simulink model "MassSpringModel"  (R2015b)
settings: Solver=ode1  StartTime=0.0  StopTime=10.0  FixedStep=0.0001  RelTol=1e-3
model workspace (MAT data in the model file):
  ans = 35
  c = 1.7
  d = 1
  g = 9.81
  m = 0.35
settings Model: Creator=aemili  LastModifiedBy=aemili

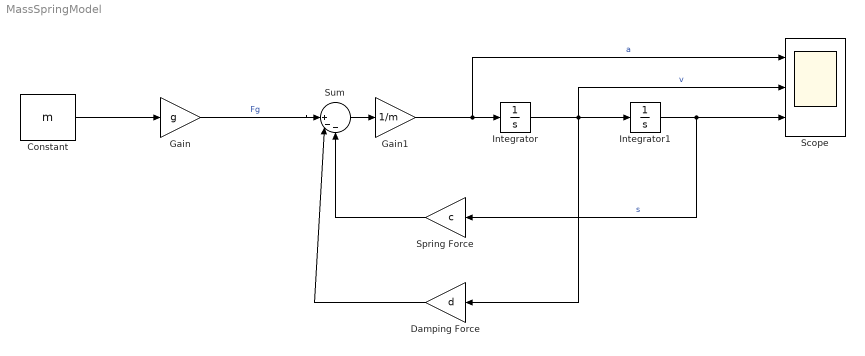
== system MassSpringModel ==
  Constant : Constant  Value=m
  Damping Force : Gain  Gain=d
  Gain : Gain  Gain=g
  Gain1 : Gain  Gain=1/m
  Integrator : Integrator
  Integrator1 : Integrator
  Scope : Scope  NumInputPorts=3
  Spring Force : Gain  Gain=c
  Sum : Sum  Inputs=||+--
  wires:
  Constant/1 -> Gain/1
  Gain/1 -> Sum/1  "Fg"
  Gain1/1 -> Scope/1, Integrator/1  "a"
  Integrator/1 -> Scope/2, Integrator1/1, Damping Force/1  "v"
  Integrator1/1 -> Spring Force/1, Scope/3  "s"
  Sum/1 -> Gain1/1
  Spring Force/1 -> Sum/3
  Damping Force/1 -> Sum/2
